simulink model "Filtro_teste"  (R2014a)
settings: Solver=ode45  StartTime=0.0  StopTime=0.04  MaxStep=1e-6  RelTol=1e-3
undefined symbols (not defined in the file or in its folder): dfilt, fdesignblkfcn, gcbh
libraries: powerlib x17, dsparch4 x1
settings Model: Creator=JPSOLIV  LastModifiedBy=Joao
settings DebuggingCC: MergeDetectMultiDrivingBlocksExec=error

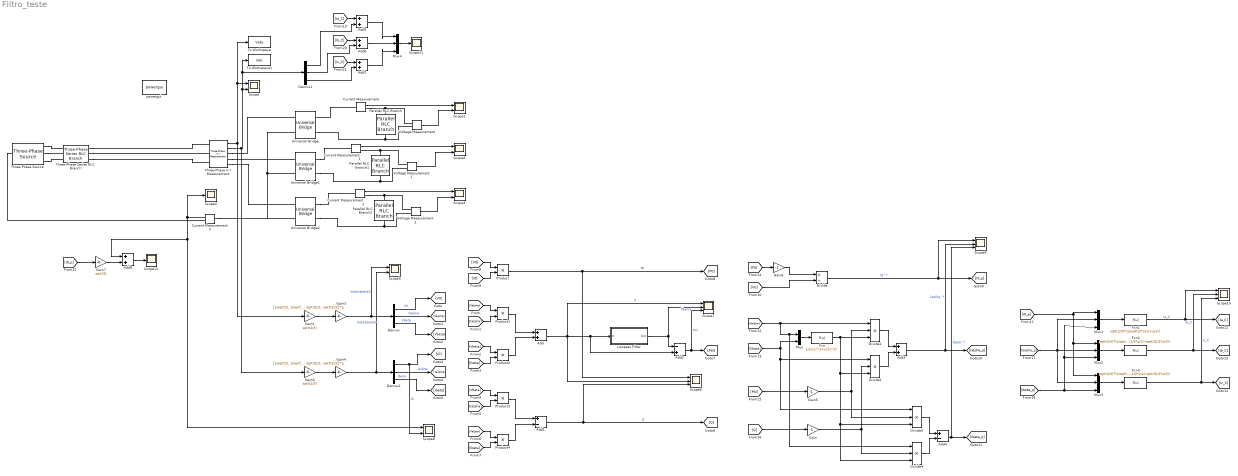
== system Filtro_teste ==
  Add{,3,5..8} (6 alike) : Sum
  Add1 : Sum  Inputs=+-
  Add2 : Sum  Inputs=-+
  Add4 : Sum  Inputs=+-
  Current Measurement{,1..3} (4 alike) : powerlib/Measurements/Current Measurement  PhasorSimulation=off  OutputType=Complex  PSBequivalent=0
  Demux : Demux  Outputs=3
  Demux1 : Demux  Outputs=3
  Demux2 : Demux  Outputs=3
  Divide : Product  Inputs=*/
  Divide{1..4} (4 alike) : Product  Inputs=***
  Fcn : Fcn  Expr=1/(u(1)^2+u(2)^2)
  Fcn1 : Fcn  Expr=sqrt(2/3)*(1/sqrt(2)*u(1)+u(2))
  Fcn2 : Fcn  Expr=sqrt(2/3)*(1/sqrt(2)*u(1)-1/2*u(2)+sqrt(3)/2*u(3))
  Fcn3 : Fcn  Expr=sqrt(2/3)*(1/sqrt(2)*u(1)-1/2*u(2)-sqrt(3)/2*u(3))
  Gain : Gain  Gain=-1
  Gain1 : Gain  Gain=sqrt(2/3)
  Gain2 : Gain  Gain=sqrt(2/3)
  Gain3 : Gain  Gain=[1/sqrt(2), 1/sqrt(2), 1/sqrt(2); 1, -1/2, -1/2; 0, sqrt(3)/2, -sqrt(3)/2]  Multiplication=Matrix(K*u)
  Gain4 : Gain  Gain=[1/sqrt(2), 1/sqrt(2), 1/sqrt(2); 1, -1/2, -1/2; 0, sqrt(3)/2, -sqrt(3)/2]  Multiplication=Matrix(K*u)
  Gain5 : Gain  Gain=-1
  Gain6 : Gain  Gain=-1
  Gain7 : Gain  Gain=sqrt(3)
  Lowpass Filter : Subsystem  DialogController=fdesignblkfcn  InitFcn=fdesignblkfcn(gcbh, {'InitFcn'});  mask(Lowpass Filter){}
      mask help: Design a lowpass filter
      settings: CopyFcn=fdesignblkfcn(gcbh, {'CopyFcn'});
      mask Help: helpview(mapfilelocation('dsp'), 'dsplowpassfilter');
      mask Display: disp('Lowpass')
  Mux : Mux  Inputs=2
  Mux{1..4} (4 alike) : Mux  Inputs=3
  Parallel RLC Branch : powerlib/Elements/Parallel RLC Branch  LConnTagsString=a  RConnTagsString=__new0  BranchType=RC  Resistance=20  Inductance=1e-3  SetiL0=off  InitialCurrent=0  Capacitance=30e-6  Setx0=off  InitialVoltage=0  Measurements=None
  Parallel RLC Branch1 : powerlib/Elements/Parallel RLC Branch  LConnTagsString=a  RConnTagsString=__new0  BranchType=RC  Resistance=20  Inductance=1e-3  SetiL0=off  InitialCurrent=0  Capacitance=30e-6  Setx0=off  InitialVoltage=0  Measurements=None
  Parallel RLC Branch2 : powerlib/Elements/Parallel RLC Branch  LConnTagsString=a  RConnTagsString=__new0  BranchType=RC  Resistance=20  Inductance=1e-3  SetiL0=off  InitialCurrent=0  Capacitance=30e-6  Setx0=off  InitialVoltage=0  Measurements=None
  Product{,1..4} (5 alike) : Product
  Scope{,1..3,5,8} (6 alike) : Scope  NumInputPorts=2
      Scope settings: YMin=-600~-200  YMax=400~200
      Scope1 settings: YMin=-0.00169333~0  YMax=20~200
      Scope2 settings: YMin=-5~-5  YMax=5~5  SaveName=ScopeData2
      Scope3 settings: YMin=-5~-5  YMax=5~5  SaveName=ScopeData3
      Scope5 settings: YMin=-600~-200  YMax=400~200  SaveName=ScopeData5
      Scope8 settings: YMin=-600~-200  YMax=400~200  SaveName=ScopeData8
  Scope{6..7,9..10} (4 alike) : Scope  NumInputPorts=3
      Scope10 settings: YMin=-600~-200~-5  YMax=400~200~5  SaveName=ScopeData10
      Scope6 settings: YMin=-600~-200~-5  YMax=400~200~5  SaveName=ScopeData6
      Scope7 settings: YMin=0~0~-5000  YMax=105000~5000~105000  SaveName=ScopeData7
      Scope9 settings: YMin=-8~-1e+12~-2.5e+14  YMax=8~2e+12~1.75e+15  SaveName=ScopeData9
  Scope11 : Scope
      settings: YMin=-600  YMax=400  SaveName=ScopeData11
  Scope12 : Scope
      settings: YMin=-7.5  YMax=7.5  SaveName=ScopeData12
  Scope4 : Scope
      settings: YMin=-25  YMax=27.5  SaveName=ScopeData4
  Three-Phase Series RLC Branch : powerlib/Elements/Three-Phase Series RLC Branch  LConnTagsString=A|B|C  RConnTagsString=A|B|C  BranchType=RL  Resistance=0.1  Inductance=1e-5  Capacitance=1e-6  Measurements=None
  Three-Phase V-I Measurement : powerlib/Measurements/Three-Phase V-I Measurement  VoltageMeasurement=phase-to-phase  SetLabelV=off  LabelV=Vabc  Vpu=off  VpuLL=off  CurrentMeasurement=yes  SetLabelI=off  LabelI=Iabc  Ipu=off  Pbase=100e6  Vbase=500e3  OutputType=Complex  PhasorSimulation=off  PSBequivalent=0
  Three-Phase Source : powerlib/Electrical Sources/Three-Phase Source  Voltage=115*sqrt(3)  PhaseAngle=0  Frequency=400  InternalConnection=Yn  SpecifyImpedance=off  Resistance=0.8929e-9  Inductance=16.58e-12  ShortCircuitLevel=100e6  BaseVoltage=115*sqrt(3)  XRratio=7  BusType=swing  Pref=0  Qref=0  Qmin=-inf  Qmax=inf
  To Workspace : ToWorkspace  VariableName=Vabc  SaveFormat=Structure With Time  SampleTime=-1
  To Workspace1 : ToWorkspace  VariableName=Iabc  SaveFormat=Structure With Time  SampleTime=-1
  Universal Bridge : powerlib/Power Electronics/Universal Bridge  Arms=2  SnubberResistance=1e5  SnubberCapacitance=inf  Device=Diodes  Ron=1e-3  Lon=0  ForwardVoltages="[  0  0  ]"  ForwardVoltage=0  GTOparameters=[ 10e-6 , 20e-6 ]  IGBTparameters=[ 1e-6 , 2e-6 ]  Measurements=None  Measurements_2=None  converterType=Rectifier
  Universal Bridge1 : powerlib/Power Electronics/Universal Bridge  Arms=2  SnubberResistance=1e5  SnubberCapacitance=inf  Device=Diodes  Ron=1e-3  Lon=0  ForwardVoltages="[  0  0  ]"  ForwardVoltage=0  GTOparameters=[ 10e-6 , 20e-6 ]  IGBTparameters=[ 1e-6 , 2e-6 ]  Measurements=None  Measurements_2=None  converterType=Rectifier
  Universal Bridge2 : powerlib/Power Electronics/Universal Bridge  Arms=2  SnubberResistance=1e5  SnubberCapacitance=inf  Device=Diodes  Ron=1e-3  Lon=0  ForwardVoltages="[  0  0  ]"  ForwardVoltage=0  GTOparameters=[ 10e-6 , 20e-6 ]  IGBTparameters=[ 1e-6 , 2e-6 ]  Measurements=None  Measurements_2=None  converterType=Rectifier
  Voltage Measurement : powerlib/Measurements/Voltage Measurement  PhasorSimulation=off  OutputType=Complex  PSBequivalent=0
  Voltage Measurement1 : powerlib/Measurements/Voltage Measurement  PhasorSimulation=off  OutputType=Complex  PSBequivalent=0
  Voltage Measurement2 : powerlib/Measurements/Voltage Measurement  PhasorSimulation=off  OutputType=Complex  PSBequivalent=0
  powergui : powerlib/powergui  Priority=1  SimulationMode=Discrete  SolverType=Tustin  SampleTime=5e-7  frequency=60  SPID=off  DisableSnubberDevices=off  DisableRonSwitches=off  DisableVfSwitches=off  SwTol=0  Interpol=off  DisplayEquations=off  Ts=100  methode=off  frequencyindice=0  Pbase=100e6  ErrMax=1e-4  Iterations=50  UnitsV=kV  UnitsW=MW  FunctionMessages=off  echomessages=off  HookPort=off  EnableUseOfTLC=off  x0status=blocks  RestoreLinks=warning  ResistiveCurrentMeasurement=off  Frange=[0:2:500]  Ylog=off  Xlog=on  ShowGrid=off  save=off  variable=ZData  structure=0  ZoomFFT=off  StartTime=0.0  cycles=1  DisplayStyle=1  fundamental=60  FreqAxis=off  MaxFrequency=1000  frequencyindicesteady=1  RmsSteady=1  display=off
  wires:
  Three-Phase V-I Measurement/1 -> To Workspace/1, Scope/1, Gain1/1
  Three-Phase V-I Measurement/2 -> Gain2/1, Demux2/1, To Workspace1/1, Scope/2
  Current Measurement/1 -> Scope1/1
  Voltage Measurement/1 -> Scope1/2
  Current Measurement1/1 -> Scope2/1
  Voltage Measurement1/1 -> Scope2/2
  Current Measurement2/1 -> Scope3/1
  Voltage Measurement2/1 -> Scope3/2
  Gain1/1 -> Gain3/1
  Gain2/1 -> Gain4/1
  Gain3/1 -> Demux/1, Scope5/1  "Valphabeta0"
  Gain4/1 -> Scope5/2, Demux1/1  "Ialphabeta0"
  Demux/1 -> [V0]  "V0"
  Product/1 -> Scope6/1, [P0]  "P0"
  Demux/2 -> [Valpha]  "Valpha"
  Demux1/2 -> [Ialpha]  "Ialpha"
  Demux/3 -> [Vbeta]  "Vbeta"
  Demux1/3 -> [Ibeta]  "Ibeta"
  Product1/1 -> Add/1
  Product2/1 -> Add/2
  Add/1 -> Scope7/1, Add2/2, Lowpass Filter/1(In), Scope6/2  "P"
  Product3/1 -> Add1/1
  Product4/1 -> Add1/2
  Add1/1 -> [Q], Scope6/3  "Q"
  Lowpass Filter/1(Out) -> Add2/1, Scope7/2  "Pbarra"
  Add2/1 -> Scope7/3, [Ptil]  "Ptil"
  Demux1/1 -> Scope8/2, [I0]  "I0"
  [Valpha] -> Product1/1
  [Ialpha] -> Product1/2
  [Vbeta] -> Product2/1
  [Ibeta] -> Product2/2
  [Vbeta] -> Product3/1
  [Ialpha] -> Product3/2
  [Valpha] -> Product4/1
  [Ibeta] -> Product4/2
  [V0] -> Product/1
  [I0] -> Product/2
  Mux/1 -> Fcn/1
  [Valpha] -> Divide4/1, Mux/1, Divide1/1
  [Vbeta] -> Mux/2, Divide2/1, Divide3/1
  [Ptil] -> Gain5/1
  Fcn/1 -> Divide4/3, Divide3/3, Divide2/3, Divide1/3
  [Q] -> Gain/1
  Divide1/1 -> Add3/1
  Divide2/1 -> Add3/2
  Divide3/1 -> Add4/1
  Divide4/1 -> Add4/2
  Add4/1 -> Scope9/3, [Ibeta_p]  "Ibeta^*"
  Add3/1 -> Scope9/2, [Ialpha_p]  "Iaplha^*"
  Divide/1 -> Scope9/1, [I0_p]  "I0^*"
  [P0] -> Gain6/1
  [V0] -> Divide/2
  Mux1/1 -> Fcn1/1
  [I0_p] -> Mux2/1, Mux3/1, Mux1/1
  [Ialpha_p] -> Mux3/2, Mux2/2, Mux1/2
  [Ibeta_p] -> Mux3/3, Mux2/3, Mux1/3
  Fcn1/1 -> [Ia_C], Scope10/1  "Ia_C"
  Mux2/1 -> Fcn2/1
  Fcn2/1 -> [Ib_C], Scope10/2  "Ib_C"
  Mux3/1 -> Fcn3/1
  Fcn3/1 -> [Ic_C], Scope10/3  "Ic_C"
  Gain/1 -> Divide2/2, Divide4/2
  Gain5/1 -> Divide1/2, Divide3/2
  Gain6/1 -> Divide/1
  [Ia_C] -> Add5/1
  [Ib_C] -> Add6/1
  [Ic_C] -> Add7/1
  Demux2/1 -> Add5/2
  Demux2/2 -> Add6/2
  Demux2/3 -> Add7/2
  Add5/1 -> Mux4/1
  Add6/1 -> Mux4/2
  Add7/1 -> Mux4/3
  Mux4/1 -> Scope11/1
  [I0_p] -> Gain7/1
  Current Measurement3/1 -> Scope4/1, Scope8/1, Add8/1
  Add8/1 -> Scope12/1
  Gain7/1 -> Add8/2
  connections:
  Universal Bridge1/LConn2 -- Current Measurement3/LConn1 -- Universal Bridge2/LConn2 -- Universal Bridge/LConn2
  Parallel RLC Branch/RConn1 -- Universal Bridge/RConn2 -- Voltage Measurement/LConn2
  Three-Phase V-I Measurement/RConn1 -- Universal Bridge/LConn1
  Three-Phase V-I Measurement/RConn2 -- Universal Bridge1/LConn1
  Three-Phase V-I Measurement/RConn3 -- Universal Bridge2/LConn1
  Current Measurement/RConn1 -- Voltage Measurement/LConn1 -- Parallel RLC Branch/LConn1
  Current Measurement/LConn1 -- Universal Bridge/RConn1
  Parallel RLC Branch1/RConn1 -- Universal Bridge1/RConn2 -- Voltage Measurement1/LConn2
  Parallel RLC Branch1/LConn1 -- Current Measurement1/RConn1 -- Voltage Measurement1/LConn1
  Universal Bridge1/RConn1 -- Current Measurement1/LConn1
  Parallel RLC Branch2/RConn1 -- Universal Bridge2/RConn2 -- Voltage Measurement2/LConn2
  Parallel RLC Branch2/LConn1 -- Current Measurement2/RConn1 -- Voltage Measurement2/LConn1
  Universal Bridge2/RConn1 -- Current Measurement2/LConn1
  Current Measurement3/RConn1 -- Three-Phase Source/LConn1
  Three-Phase Source/RConn1 -- Three-Phase Series RLC Branch/LConn1
  Three-Phase Source/RConn2 -- Three-Phase Series RLC Branch/LConn2
  Three-Phase Source/RConn3 -- Three-Phase Series RLC Branch/LConn3
  Three-Phase Series RLC Branch/RConn2 -- Three-Phase V-I Measurement/LConn2
  Three-Phase Series RLC Branch/RConn1 -- Three-Phase V-I Measurement/LConn1
  Three-Phase Series RLC Branch/RConn3 -- Three-Phase V-I Measurement/LConn3

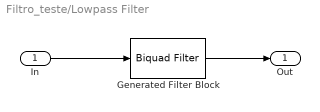
== system Filtro_teste/Lowpass Filter ==
  In : Inport
  Generated Filter Block : dsparch4/Biquad Filter  Tag=BlockMethodSubSystem  IIRFiltStruct=Direct form II  CoeffSource=Specify via dialog  BiQuadCoeffs=[1.9581181503870373e-08 3.9162363007740746e-08 1.9581181503870373e-08 1 -1.999872600061211 0.99987271195891581;0.24151271759227033 0.48302543518454066 0.24151271759227033 1 -1.9996926850262837 0.99969272713599988]  a0Flag=Warning  IC=0  ICnum=0  ICden=0  InputProcessing=Columns as channels (frame based)  denAccumFracLength=30  denProdOutputFracLength=30  secondMemoryFracLength=15  roundingMode=Floor  overflowMode=off  ScaleValues=[6.0159553970087562e-08;1;1]  optimizeScaleValues=off  ScaleValueMode=Specify via input port (g)  scaleValueFracLength=14  FilterSource=Specify via dialog  dfiltObjectName=dfilt.df2tsos([1 0.3 0.4],[1 0.1 0.2])
  Out : Outport
  wires:
  In/1 -> Generated Filter Block/1
  Generated Filter Block/1 -> Out/1
